simulink model "elec3200lab4"  (R2016a)
settings: Solver=VariableStepAuto  StartTime=0.0  StopTime=20.0  RelTol=1e-3
settings Model: Creator=古乔  LastModifiedBy=古乔

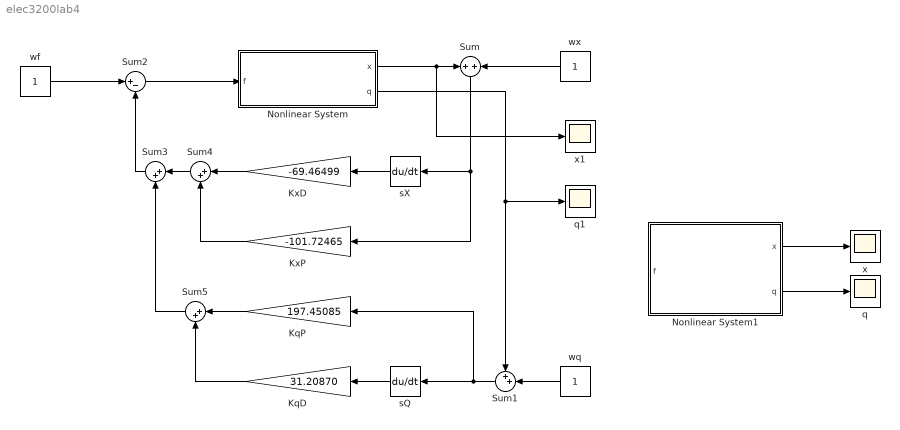
== system elec3200lab4 ==
  KqD : Gain  Gain=31.20870
  KqP : Gain  Gain=197.45085
  KxD : Gain  Gain=-69.46499
  KxP : Gain  Gain=-101.72465
  Nonlinear System : Subsystem
  Nonlinear System1 : Subsystem
  Sum : Sum  Inputs=+|+
  Sum1 : Sum  Inputs=++|
  Sum2 : Sum  Inputs=|+-
  Sum3 : Sum  Inputs=|++
  Sum4 : Sum  Inputs=|++
  Sum5 : Sum  Inputs=|++
  q : Scope
  q1 : Scope
  sQ : Derivative
  sX : Derivative
  wf : Constant
  wq : Constant
  wx : Constant
  x : Scope
  x1 : Scope
  wires:
  Nonlinear System/1(x) -> x1/1, Sum/1
  Nonlinear System/2(q) -> Sum1/1, q1/1
  wx/1 -> Sum/2
  wq/1 -> Sum1/2
  Sum2/1 -> Nonlinear System/1(f)
  wf/1 -> Sum2/1
  Sum/1 -> KxP/1, sX/1
  Sum1/1 -> KqP/1, sQ/1
  Sum4/1 -> Sum3/1
  Sum5/1 -> Sum3/2
  Sum3/1 -> Sum2/2
  sQ/1 -> KqD/1
  sX/1 -> KxD/1
  KqP/1 -> Sum5/1
  KqD/1 -> Sum5/2
  KxD/1 -> Sum4/1
  KxP/1 -> Sum4/2
  Nonlinear System1/2(q) -> q/1
  Nonlinear System1/1(x) -> x/1

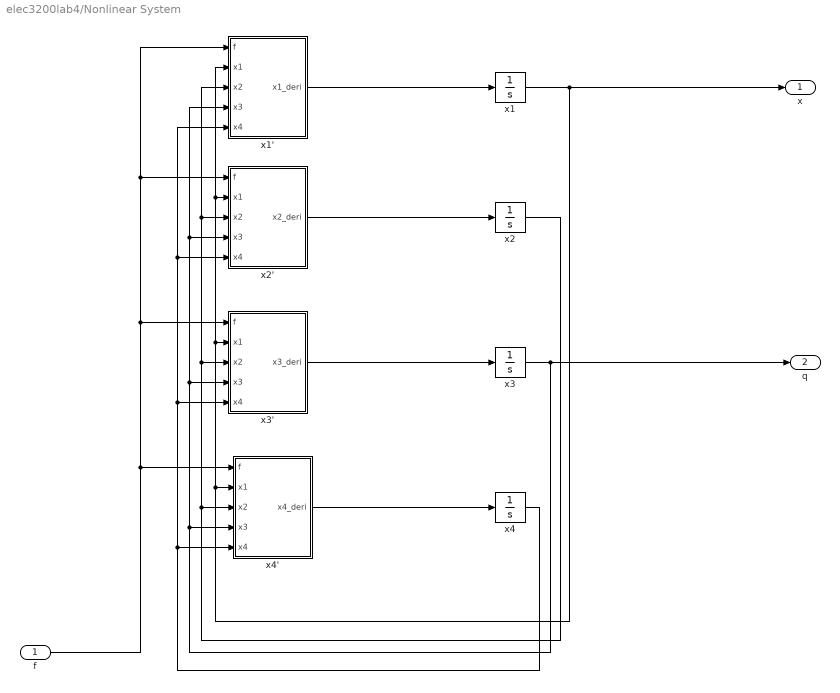
== system elec3200lab4/Nonlinear System ==
  f : Inport
  x1 : Integrator  InitialCondition=-0.3
  x1' : MATLAB Function  TreatAsAtomicUnit=on
  x2 : Integrator
  x2' : MATLAB Function  TreatAsAtomicUnit=on
  x3 : Integrator  InitialCondition=-5/180*pi
  x3' : MATLAB Function  TreatAsAtomicUnit=on
  x4 : Integrator  InitialCondition=-0.5
  x4' : MATLAB Function  TreatAsAtomicUnit=on
  x : Outport
  q : Outport  Port=2
  wires:
  f/1 -> x4'/1(f), x3'/1(f), x2'/1(f), x1'/1(f)
  x1'/1(x1_deri) -> x1/1
  x4'/1(x4_deri) -> x4/1
  x3'/1(x3_deri) -> x3/1
  x2'/1(x2_deri) -> x2/1
  x1/1 -> x1'/2(x1), x2'/2(x1), x3'/2(x1), x4'/2(x1), x/1
  x2/1 -> x3'/3(x2), x1'/3(x2), x2'/3(x2), x4'/3(x2)
  x3/1 -> q/1, x1'/4(x3), x2'/4(x3), x3'/4(x3), x4'/4(x3)
  x4/1 -> x1'/5(x4), x2'/5(x4), x3'/5(x4), x4'/5(x4)

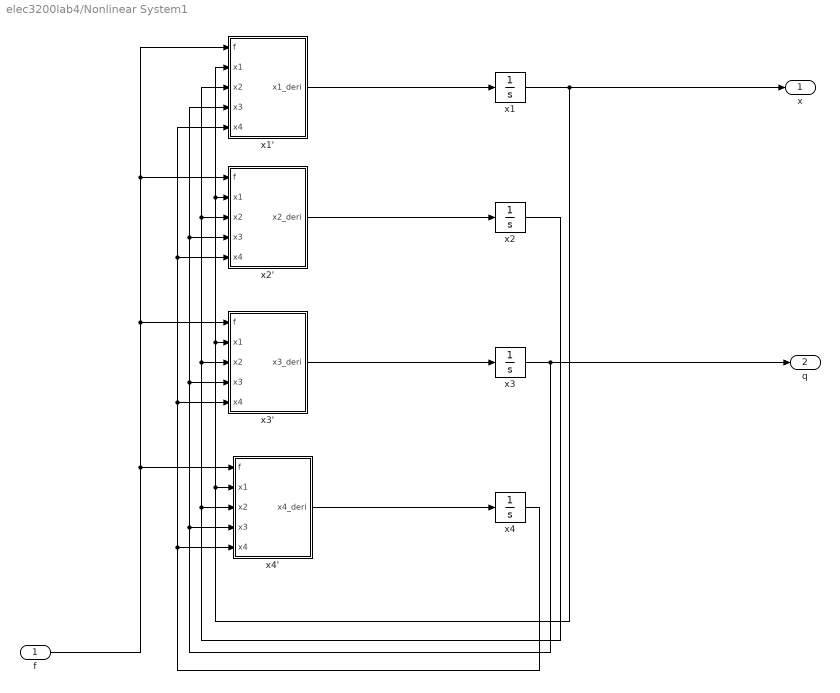
== system elec3200lab4/Nonlinear System1 ==
  f : Inport
  x1 : Integrator
  x1' : MATLAB Function  TreatAsAtomicUnit=on
  x2 : Integrator
  x2' : MATLAB Function  TreatAsAtomicUnit=on
  x3 : Integrator  InitialCondition=3/180*pi
  x3' : MATLAB Function  TreatAsAtomicUnit=on
  x4 : Integrator
  x4' : MATLAB Function  TreatAsAtomicUnit=on
  x : Outport
  q : Outport  Port=2
  wires:
  f/1 -> x4'/1(f), x3'/1(f), x2'/1(f), x1'/1(f)
  x1'/1(x1_deri) -> x1/1
  x4'/1(x4_deri) -> x4/1
  x3'/1(x3_deri) -> x3/1
  x2'/1(x2_deri) -> x2/1
  x1/1 -> x1'/2(x1), x2'/2(x1), x3'/2(x1), x4'/2(x1), x/1
  x2/1 -> x3'/3(x2), x1'/3(x2), x2'/3(x2), x4'/3(x2)
  x3/1 -> q/1, x1'/4(x3), x2'/4(x3), x3'/4(x3), x4'/4(x3)
  x4/1 -> x1'/5(x4), x2'/5(x4), x3'/5(x4), x4'/5(x4)

== matlab function elec3200lab4/Nonlinear System/x2' ==
  data: f input; x1 input; x2_deri output; x2 input; x3 input; x4 input
function x2_deri  = cal_dx2(f,x1,x2,x3,x4)
Mp = 0.07;
Mc = 1.42;
Mb = 0.05;
g = 9.8;
L = 0.335;

x2_deri = (- 12*L*sin(x3)*Mb^2*x4^2 + 12*g*cos(x3)*sin(x3)*Mb^2 - 10*L*sin(x3)*Mb*Mp*x4^2 + 12*g*cos(x3)*sin(x3)*Mb*Mp ...
    + 12*f*Mb - 2*L*sin(x3)*Mp^2*x4^2 + 3*g*cos(x3)*sin(x3)*Mp^2 + 4*f*Mp)...
    /(12*Mb^2 - 3*Mp^2*cos(x3)^2 - 12*Mb^2*cos(x3)^2 + 4*Mp^2 + 12*Mb*Mc + 16*Mb*Mp + 4*Mc*Mp - 12*Mb*Mp*cos(x3)^2);

== matlab function elec3200lab4/Nonlinear System/x3' ==
  data: f input; x1 input; x3_deri output; x2 input; x3 input; x4 input
function x3_deri  = cal_dx3(f,x1,x2,x3,x4)
Mp = 0.07;
Mc = 1.42;
Mb = 0.05;
g = 9.8;
L = 0.335;

x3_deri = x4;

== matlab function elec3200lab4/Nonlinear System/x1' ==
  data: f input; x1 input; x1_deri output; x2 input; x3 input; x4 input
function x1_deri  = cal_dx1(f,x1,x2,x3,x4)
Mp = 0.07;
Mc = 1.42;
Mb = 0.05;
g = 9.8;
L = 0.335;

x1_deri = x2;

== matlab function elec3200lab4/Nonlinear System/x4' ==
  data: f input; x1 input; x4_deri output; x2 input; x3 input; x4 input
function x4_deri  = cal_dx4(f,x1,x2,x3,x4)
Mp = 0.07;
Mc = 1.42;
Mb = 0.05;
g = 9.8;
L = 0.335;

x4_deri = (3*(2*Mb + Mp)*(2*f*cos(x3) + 2*Mb*g*sin(x3) + 2*Mc*g*sin(x3) + 2*Mp*g*sin(x3) - 2*L*Mb*x4^2*cos(x3)*sin(x3) - L*Mp*x4^2*cos(x3)*sin(x3)))...
    /(L*(12*Mb^2 - 3*Mp^2*cos(x3)^2 - 12*Mb^2*cos(x3)^2 + 4*Mp^2 + 12*Mb*Mc + 16*Mb*Mp + 4*Mc*Mp - 12*Mb*Mp*cos(x3)^2));

== matlab function elec3200lab4/Nonlinear System1/x1' ==
  data: f input; x1 input; x1_deri output; x2 input; x3 input; x4 input
function x1_deri  = cal_dx1(f,x1,x2,x3,x4)
Mp = 0.07;
Mc = 1.42;
Mb = 0.05;
g = 9.8;
L = 0.335;

x1_deri = x2;

== matlab function elec3200lab4/Nonlinear System1/x2' ==
  data: f input; x1 input; x2_deri output; x2 input; x3 input; x4 input
function x2_deri  = cal_dx2(f,x1,x2,x3,x4)
Mp = 0.07;
Mc = 1.42;
Mb = 0.05;
g = 9.8;
L = 0.335;

x2_deri = (- 12*L*sin(x3)*Mb^2*x4^2 + 12*g*cos(x3)*sin(x3)*Mb^2 - 10*L*sin(x3)*Mb*Mp*x4^2 + 12*g*cos(x3)*sin(x3)*Mb*Mp + 12*f*Mb - 2*L*sin(x3)*Mp^2*x4^2 + 3*g*cos(x3)*sin(x3)*Mp^2 + 4*f*Mp)...
    /(12*Mb^2 - 3*Mp^2*cos(x3)^2 - 12*Mb^2*cos(x3)^2 + 4*Mp^2 + 12*Mb*Mc + 16*Mb*Mp + 4*Mc*Mp - 12*Mb*Mp*cos(x3)^2);

== matlab function elec3200lab4/Nonlinear System1/x3' ==
  data: f input; x1 input; x3_deri output; x2 input; x3 input; x4 input
function x3_deri  = cal_dx3(f,x1,x2,x3,x4)
Mp = 0.07;
Mc = 1.42;
Mb = 0.05;
g = 9.8;
L = 0.335;

x3_deri = x4;

== matlab function elec3200lab4/Nonlinear System1/x4' ==
  data: f input; x1 input; x4_deri output; x2 input; x3 input; x4 input
function x4_deri  = cal_dx4(f,x1,x2,x3,x4)
Mp = 0.07;
Mc = 1.42;
Mb = 0.05;
g = 9.8;
L = 0.335;

x4_deri = (3*(2*Mb + Mp)*(2*f*cos(x3) + 2*Mb*g*sin(x3) + 2*Mc*g*sin(x3) + 2*Mp*g*sin(x3) - 2*L*Mb*x4^2*cos(x3)*sin(x3) - L*Mp*x4^2*cos(x3)*sin(x3)))...
    /(L*(12*Mb^2 - 3*Mp^2*cos(x3)^2 - 12*Mb^2*cos(x3)^2 + 4*Mp^2 + 12*Mb*Mc + 16*Mb*Mp + 4*Mc*Mp - 12*Mb*Mp*cos(x3)^2));
